simulink model "realtimeBalrob"  (R2024b)
settings: Solver=FixedStepDiscrete  StartTime=0.0  StopTime=50  FixedStep=0.01  RelTol=1e-3  EnableMultiTasking=on
undefined symbols (not defined in the file): chassis, DiscIntNeverNeededParam, Discrete, drv, feedback, filter, gbox, sens, sIn, Time, wheel
libraries: BalRobTbx_baselib x9, simulink x3, ctrlSharedLib x1
settings Model: ExtModeTrigDuration=2  Creator=priesmaxim  LastModifiedBy=priesmaxim
settings SolverCC: AutoInsertRateTranBlk=on
settings OptimizationCC: EnhancedBackFolding=on  PassReuseOutputArgsAs=Individual arguments  ZeroExternalMemoryAtStartup=off  ZeroInternalMemoryAtStartup=off  MaxStackSize=64  OptimizeBlockOrder=speed  DifferentSizesBufferReuse=on  OptimizationCustomize=off  EfficientTunableParamExpr=on
settings DebuggingCC: ParameterTunabilityLossMsg=error
settings HardwareCC: ProdBitPerInt=16  ProdBitPerPointer=16  ProdBitPerSizeT=16  ProdBitPerPtrDiffT=16  ProdLargestAtomicFloat=None  ProdWordSize=8  ProdHWDeviceType=Atmel->AVR
settings SFSimCC: MATLABDynamicMemAlloc=off
settings RTWCC: Description=Embedded Coder  SystemTargetFile=ert.tlc  HardwareBoard=Arduino Mega 2560  TemplateMakefile=ert_default_tmf  Toolchain=Arduino AVR  BuildConfiguration=Faster Runs
settings CodeAppCC: ForceParamTrailComments=on  IgnoreCustomStorageClasses=off  OperatorAnnotations=on  SimulinkDataObjDesc=on  SFDataObjDesc=on  InsertBlockDesc=on
settings ERTTargetCC: SupportContinuousTime=on  SupportVariableSizeSignals=on  ExtModeTransport=3  ExtModeStaticAlloc=on  ExtModeAutomaticAllocSize=off  ExtModeStaticAllocSize=2048  ExtModeMexFile=ext_xcp  ExtModeIntrfLevel=Level2 - Open  InlinedParameterPlacement=Hierarchical

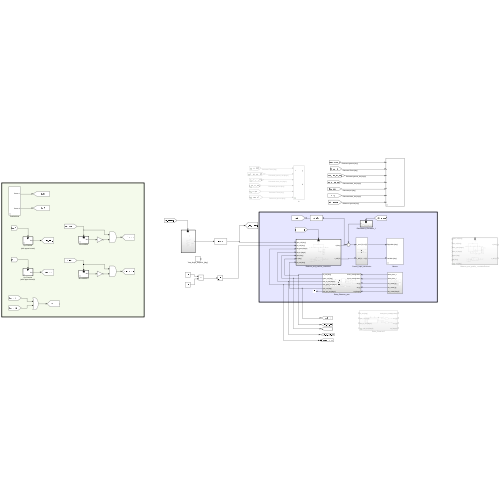
[thumbnail: Simulink's stored preview of the top-level diagram]
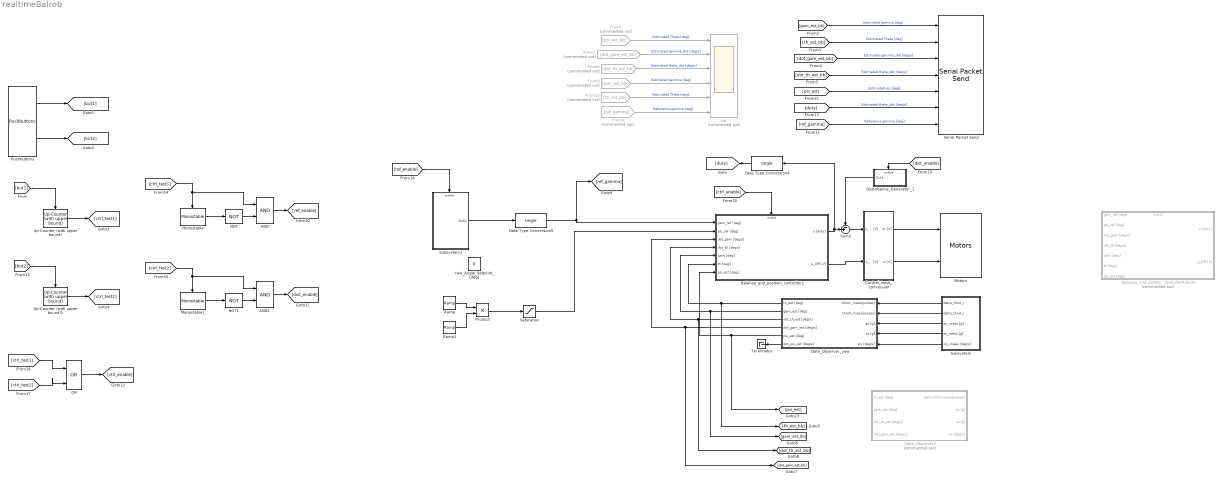
== system realtimeBalrob ==
  AND : Logic  IconShape=distinctive  AllPortsSameDT=off  OutDataTypeStr=boolean
  AND1 : Logic  IconShape=distinctive  AllPortsSameDT=off  OutDataTypeStr=boolean
  Balance_and_positio_ controllerRobust : Subsystem  Commented=on
  Balance_and_position_controller1 : Subsystem
  Control_Input_conversion : Subsystem
  Data Type Conversion4 : DataTypeConversion  OutDataTypeStr=single  SaturateOnIntegerOverflow=off  RndMeth=Floor
  Data Type Conversion5 : DataTypeConversion  OutDataTypeStr=single  SaturateOnIntegerOverflow=off  RndMeth=Floor
  Disturbance_Generator_1 : Subsystem  TreatAsAtomicUnit=on
  From1 : From  Commented=on  GotoTag=psi_est_bb
  From10 : From  Commented=on  GotoTag=th_est_bb
  From6 : From  Commented=on  GotoTag=ref_gamma
  From7 : From  Commented=on  GotoTag=dot_gam_est_bb
  From8 : From  Commented=on  GotoTag=dot_th_est_bb
  From9 : From  Commented=on  GotoTag=gam_est_bb
  Monostable : BalRobTbx_baselib/Utilities/Monostable  Tp=1
      settings: SourceProductName=Balancing Robot Toolbox
  Monostable1 : BalRobTbx_baselib/Utilities/Monostable  Tp=1
      settings: SourceProductName=Balancing Robot Toolbox
  Motors : BalRobTbx_baselib/Outputs/Motors
      settings: SourceProductName=Balancing Robot Toolbox
  NOT : Logic  Operator=NOT  IconShape=distinctive  AllPortsSameDT=off  OutDataTypeStr=boolean
  NOT1 : Logic  Operator=NOT  IconShape=distinctive  AllPortsSameDT=off  OutDataTypeStr=boolean
  OR : Logic  Operator=OR  IconShape=distinctive  AllPortsSameDT=off  OutDataTypeStr=boolean
  Product : Product
  Pushbuttons : BalRobTbx_baselib/Inputs/Pushbuttons
      settings: SourceProductName=Balancing Robot Toolbox
  Ramp : simulink/Sources/Ramp  slope=100  start=0  InitialOutput=0
  Ramp1 : simulink/Sources/Ramp  slope=100  start=0  InitialOutput=0
  Saturation : Saturate  UpperLimit=500  LowerLimit=0
  Serial Packet Send : BalRobTbx_baselib/Communication/Serial Packet Send  serialLinkOpt=Bluetooth  baudRateOpt=38400  waitHostTxCmd=on  txStartCmd=65  txStopCmd=66  packetSpec={'single', 'single', 'single', 'single', 'single', 'single', 'single'}  cobsEncoded=on  nullTerminated=on  showEnablePort=off
      settings: SourceProductName=Balancing Robot Toolbox
  State_Observer2 : Subsystem  Commented=on
  State_Observer_yaw : Subsystem
  Subsystem : Subsystem
  Subsystem1 : Subsystem
  Sum2 : Sum  Inputs=-+|
  Terminator : Terminator
  Up-Counter (with upper bound) : BalRobTbx_baselib/Utilities/Up-Counter (with upper bound)  CMAX=1  C0=0
      settings: SourceProductName=Balancing Robot Toolbox
  Up-Counter (with upper bound)1 : BalRobTbx_baselib/Utilities/Up-Counter (with upper bound)  CMAX=1  C0=0
      settings: SourceProductName=Balancing Robot Toolbox
  Yaw_Angle_Setpoint_[deg] : Constant  Value=0
  bb : Scope  Commented=on  NumInputPorts=6
  wires:
  Control_Input_conversion/1(ur [V]) -> Motors/1
  Sum2/1 -> Control_Input_conversion/1(u_sum [V])
  From10/1 -> bb/5  "Estimated Theta [deg]"
  Disturbance_Generator_1/1(Out1) -> Sum2/1
  From8/1 -> bb/3  "Estimated theta_dot [deg/s]"
  From1/1 -> bb/1  "Estimated Theta [deg]"
  Control_Input_conversion/2(ul [V]) -> Motors/2
  From6/1 -> bb/6  "Reference gamma [deg]"
  From9/1 -> bb/4  "Estimated gamma [deg]"
  [dist_enable] -> Disturbance_Generator_1/Enable
  From7/1 -> bb/2  "Estimated gamma_dot [deg/s]"
  State_Observer_yaw/1(th_est [deg]) -> Balance_and_position_controller1/6(th [deg]), [th_est_bb]
  State_Observer_yaw/2(gam_est [deg]) -> Balance_and_position_controller1/5(gam [deg]), [gam_est_bb]
  State_Observer_yaw/3(dot_th_est [deg/s]) -> Balance_and_position_controller1/4(dot_th [deg/s]), [dot_th_est_bb]
  State_Observer_yaw/4(dot_gam_est [deg/s]) -> [dot_gam_est_bb], Balance_and_position_controller1/3(dot_gam [deg/s])
  [gam_est_bb] -> Serial Packet Send/1  "Estimated gamma [deg]"
  [th_est_bb] -> Serial Packet Send/2  "Estimated Theta [deg]"
  [dot_gam_est_bb] -> Serial Packet Send/3  "Estimated gamma_dot [deg/s]"
  [dot_th_est_bb] -> Serial Packet Send/4  "Estimated theta_dot [deg/s]"
  Data Type Conversion5/1 -> Balance_and_position_controller1/1(gam_ref [deg]), [ref_gamma]
  Data Type Conversion4/1 -> [duty]
  Pushbuttons/1 -> [but1]
  Pushbuttons/2 -> [but2]
  [but1] -> Up-Counter (with upper bound)/Trigger
  Up-Counter (with upper bound)/1 -> [ctrl_test1]
  [but2] -> Up-Counter (with upper bound)1/Trigger
  Up-Counter (with upper bound)1/1 -> [ctrl_test2]
  [ctrl_test1] -> Monostable/Enable, AND/1
  Monostable/1 -> NOT/1
  NOT/1 -> AND/2
  AND/1 -> [ref_enable]
  AND1/1 -> [dist_enable]
  NOT1/1 -> AND1/2
  Monostable1/1 -> NOT1/1
  [ctrl_test2] -> AND1/1, Monostable1/Enable
  [ctrl_test1] -> OR/1
  [ctrl_test2] -> OR/2
  OR/1 -> [ctrl_enable]
  Subsystem1/1(Out1) -> Data Type Conversion5/1
  [ref_enable] -> Subsystem1/Enable
  State_Observer_yaw/6(dot_psi_est [deg/s]) -> Terminator/1
  State_Observer_yaw/5(psi_est [deg]) -> Balance_and_position_controller1/7(psi_est [deg]), [psi_est]
  Subsystem/5(wy_meas [deg/s]) -> State_Observer_yaw/5(wy [deg/s])
  Subsystem/4(az_meas [g]) -> State_Observer_yaw/4(az [g])
  Subsystem/3(ax_meas [g]) -> State_Observer_yaw/3(ax [g])
  Subsystem/2(delta_throt_l) -> State_Observer_yaw/2(throtl_meas[pulses])
  Subsystem/1(delta_throt_r) -> State_Observer_yaw/1(throtr_meas[pulses])
  [duty] -> Serial Packet Send/6  "Estimated theta_dot [deg/s]"
  [ref_gamma] -> Serial Packet Send/7  "Reference gamma [deg]"
  [psi_est] -> Serial Packet Send/5  "Estimated psi [deg]"
  [ctrl_enable] -> Balance_and_position_controller1/Enable
  Balance_and_position_controller1/1(u [duty]) -> Data Type Conversion4/1, Sum2/2
  Balance_and_position_controller1/2(u_diff [V]) -> Control_Input_conversion/2(u_diff [V])
  Ramp/1 -> Product/1
  Ramp1/1 -> Product/2
  Product/1 -> Saturation/1
  Saturation/1 -> Balance_and_position_controller1/2(psi_ref [deg])

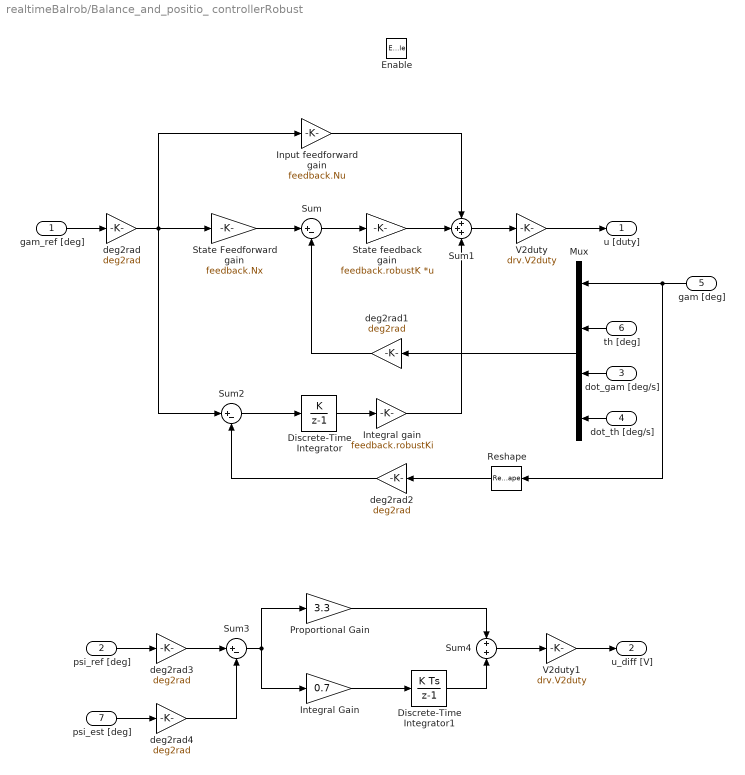
== system realtimeBalrob/Balance_and_positio_ controllerRobust ==
  gam_ref [deg] : Inport
  psi_ref [deg] : Inport  Port=2
  dot_gam [deg/s] : Inport  Port=3
  dot_th [deg/s] : Inport  Port=4
  gam [deg] : Inport  Port=5
  th [deg] : Inport  Port=6
  psi_est [deg] : Inport  Port=7
  Enable : EnablePort
  Discrete-Time Integrator : DiscreteIntegrator  IntegratorMethod=Accumulation: Forward Euler  SampleTime=sIn.Ts  ICPrevOutput=DiscIntNeverNeededParam  ICPrevScaledInput=DiscIntNeverNeededParam
  Discrete-Time Integrator1 : DiscreteIntegrator  SampleTime=-1  ICPrevOutput=DiscIntNeverNeededParam  ICPrevScaledInput=DiscIntNeverNeededParam
  Input feedforward gain : Gain  Gain=feedback.Nu
  Integral Gain : Gain  Gain=0.7
  "Integral gain " : Gain  Gain=feedback.robustKi
  Mux : Mux
  Proportional Gain : Gain  Gain=3.3
  Reshape : Reshape  OutputDimensionality=Customize  OutputDimensions=1
  State Feedforward gain : Gain  Gain=feedback.Nx
  State feedback gain : Gain  Gain=feedback.robustK  Multiplication=Matrix(K*u)
  Sum : Sum  Inputs=|+-
  Sum1 : Sum  Inputs=+++
  Sum2 : Sum  Inputs=|+-
  Sum3 : Sum  Inputs=|+-
  Sum4 : Sum  Inputs=+|+
  V2duty : Gain  Gain=drv.V2duty
  V2duty1 : Gain  Gain=drv.V2duty
  deg2rad{,1..4} (5 alike) : Gain  Gain=deg2rad
  u [duty] : Outport  OutputWhenDisabled=reset  InitialOutput=0
  u_diff [V] : Outport  Port=2  OutputWhenDisabled=reset  InitialOutput=0
  wires:
  gam_ref [deg]/1 -> deg2rad/1
  State Feedforward gain/1 -> Sum/1
  deg2rad1/1 -> Sum/2
  Mux/1 -> deg2rad1/1
  dot_th [deg/s]/1 -> Mux/4
  dot_gam [deg/s]/1 -> Mux/3
  th [deg]/1 -> Mux/2
  Sum/1 -> State feedback gain/1
  State feedback gain/1 -> Sum1/2
  Input feedforward gain/1 -> Sum1/1
  Sum1/1 -> V2duty/1
  V2duty/1 -> u [duty]/1
  Sum2/1 -> Discrete-Time Integrator/1
  deg2rad2/1 -> Sum2/2
  deg2rad/1 -> Sum2/1, Input feedforward gain/1, State Feedforward gain/1
  gam [deg]/1 -> Reshape/1, Mux/1
  Discrete-Time Integrator/1 -> "Integral gain "/1
  Reshape/1 -> deg2rad2/1
  "Integral gain "/1 -> Sum1/3
  Integral Gain/1 -> Discrete-Time Integrator1/1
  Proportional Gain/1 -> Sum4/1
  Sum3/1 -> Integral Gain/1, Proportional Gain/1
  deg2rad3/1 -> Sum3/1
  deg2rad4/1 -> Sum3/2
  Discrete-Time Integrator1/1 -> Sum4/2
  V2duty1/1 -> u_diff [V]/1
  psi_ref [deg]/1 -> deg2rad3/1
  Sum4/1 -> V2duty1/1
  psi_est [deg]/1 -> deg2rad4/1

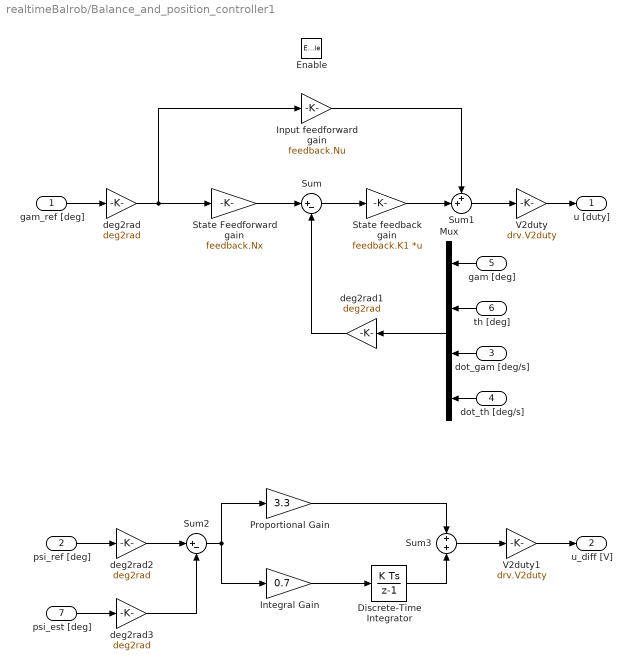
== system realtimeBalrob/Balance_and_position_controller1 ==
  gam_ref [deg] : Inport
  psi_ref [deg] : Inport  Port=2
  dot_gam [deg/s] : Inport  Port=3
  dot_th [deg/s] : Inport  Port=4
  gam [deg] : Inport  Port=5
  th [deg] : Inport  Port=6
  psi_est [deg] : Inport  Port=7
  Enable : EnablePort
  Discrete-Time Integrator : DiscreteIntegrator  SampleTime=-1  ICPrevOutput=DiscIntNeverNeededParam  ICPrevScaledInput=DiscIntNeverNeededParam
  Input feedforward gain : Gain  Gain=feedback.Nu
  Integral Gain : Gain  Gain=0.7
  Mux : Mux
  Proportional Gain : Gain  Gain=3.3
  State Feedforward gain : Gain  Gain=feedback.Nx
  State feedback gain : Gain  Gain=feedback.K1  Multiplication=Matrix(K*u)
  Sum : Sum  Inputs=|+-
  Sum1 : Sum  Inputs=++|
  Sum2 : Sum  Inputs=|+-
  Sum3 : Sum  Inputs=+|+
  V2duty : Gain  Gain=drv.V2duty
  V2duty1 : Gain  Gain=drv.V2duty
  deg2rad{,1..3} (4 alike) : Gain  Gain=deg2rad
  u [duty] : Outport  OutputWhenDisabled=reset  InitialOutput=0
  u_diff [V] : Outport  Port=2  OutputWhenDisabled=reset  InitialOutput=0
  wires:
  gam_ref [deg]/1 -> deg2rad/1
  deg2rad/1 -> Input feedforward gain/1, State Feedforward gain/1
  State Feedforward gain/1 -> Sum/1
  deg2rad1/1 -> Sum/2
  Mux/1 -> deg2rad1/1
  gam [deg]/1 -> Mux/1
  dot_th [deg/s]/1 -> Mux/4
  dot_gam [deg/s]/1 -> Mux/3
  th [deg]/1 -> Mux/2
  Sum/1 -> State feedback gain/1
  State feedback gain/1 -> Sum1/2
  Input feedforward gain/1 -> Sum1/1
  Sum1/1 -> V2duty/1
  V2duty/1 -> u [duty]/1
  psi_ref [deg]/1 -> deg2rad2/1
  psi_est [deg]/1 -> deg2rad3/1
  deg2rad2/1 -> Sum2/1
  deg2rad3/1 -> Sum2/2
  Integral Gain/1 -> Discrete-Time Integrator/1
  Sum2/1 -> Integral Gain/1, Proportional Gain/1
  Proportional Gain/1 -> Sum3/1
  Discrete-Time Integrator/1 -> Sum3/2
  Sum3/1 -> V2duty1/1
  V2duty1/1 -> u_diff [V]/1

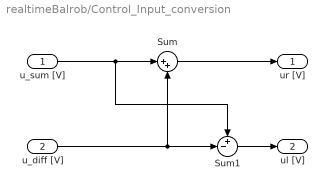
== system realtimeBalrob/Control_Input_conversion ==
  u_sum [V] : Inport
  u_diff [V] : Inport  Port=2
  Sum : Sum  Inputs=|++
  Sum1 : Sum  Inputs=+-|
  ur [V] : Outport
  ul [V] : Outport  Port=2
  wires:
  u_sum [V]/1 -> Sum/1, Sum1/1
  Sum/1 -> ur [V]/1
  u_diff [V]/1 -> Sum/2, Sum1/2
  Sum1/1 -> ul [V]/1

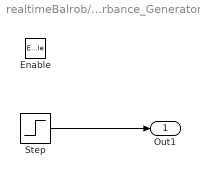
== system realtimeBalrob/Disturbance_Generator_1 ==
  Enable : EnablePort
  Step : Step  Time=10  After=5/drv.duty2V  SampleTime=0
  Out1 : Outport  OutputWhenDisabled=reset  InitialOutput=0
  wires:
  Step/1 -> Out1/1

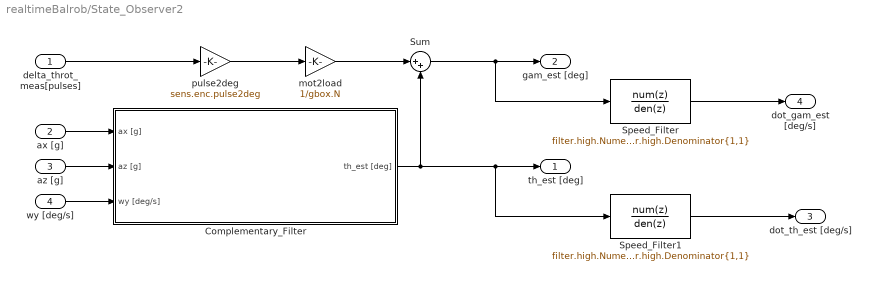
== system realtimeBalrob/State_Observer2 ==
  delta_throt_meas[pulses] : Inport
  ax [g] : Inport  Port=2
  az [g] : Inport  Port=3
  wy [deg/s] : Inport  Port=4
  Complementary_Filter : Subsystem
  Speed_Filter : DiscreteFilter  Numerator=filter.high.Numerator{1,1}  Denominator=filter.high.Denominator{1,1}
  Speed_Filter1 : DiscreteFilter  Numerator=filter.high.Numerator{1,1}  Denominator=filter.high.Denominator{1,1}
  Sum : Sum  Inputs=|++
  mot2load : Gain  Gain=1/gbox.N
  pulse2deg : Gain  Gain=sens.enc.pulse2deg
  th_est [deg] : Outport
  gam_est [deg] : Outport  Port=2
  dot_th_est [deg/s] : Outport  Port=3
  dot_gam_est [deg/s] : Outport  Port=4
  wires:
  wy [deg/s]/1 -> Complementary_Filter/3(wy [deg/s])
  az [g]/1 -> Complementary_Filter/2(az [g])
  ax [g]/1 -> Complementary_Filter/1(ax [g])
  Complementary_Filter/1(th_est [deg]) -> Sum/2, Speed_Filter1/1, th_est [deg]/1
  delta_throt_meas[pulses]/1 -> pulse2deg/1
  pulse2deg/1 -> mot2load/1
  mot2load/1 -> Sum/1
  Sum/1 -> Speed_Filter/1, gam_est [deg]/1
  Speed_Filter1/1 -> dot_th_est [deg/s]/1
  Speed_Filter/1 -> dot_gam_est [deg/s]/1

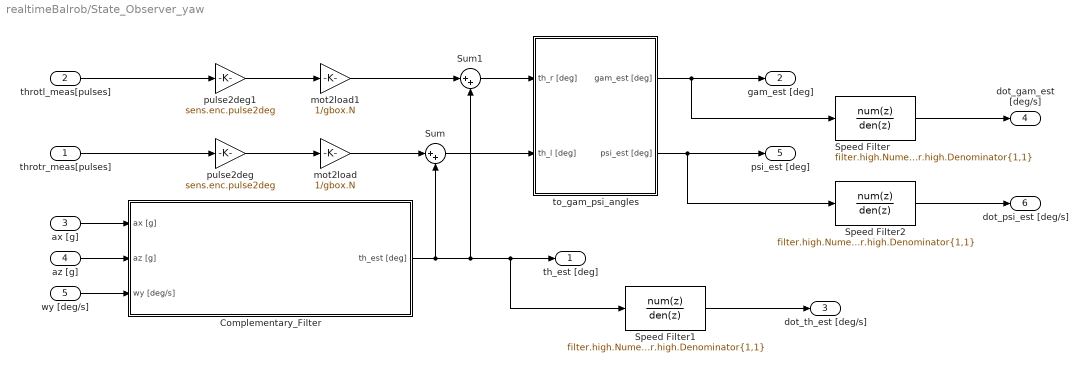
== system realtimeBalrob/State_Observer_yaw ==
  throtr_meas[pulses] : Inport
  throtl_meas[pulses] : Inport  Port=2
  ax [g] : Inport  Port=3
  az [g] : Inport  Port=4
  wy [deg/s] : Inport  Port=5
  Complementary_Filter : Subsystem
  Speed Filter : DiscreteFilter  Numerator=filter.high.Numerator{1,1}  Denominator=filter.high.Denominator{1,1}
  Speed Filter1 : DiscreteFilter  Numerator=filter.high.Numerator{1,1}  Denominator=filter.high.Denominator{1,1}
  Speed Filter2 : DiscreteFilter  Numerator=filter.high.Numerator{1,1}  Denominator=filter.high.Denominator{1,1}
  Sum : Sum  Inputs=|++
  Sum1 : Sum  Inputs=|++
  mot2load : Gain  Gain=1/gbox.N
  mot2load1 : Gain  Gain=1/gbox.N
  pulse2deg : Gain  Gain=sens.enc.pulse2deg
  pulse2deg1 : Gain  Gain=sens.enc.pulse2deg
  to_gam_psi_angles : Subsystem
  th_est [deg] : Outport
  gam_est [deg] : Outport  Port=2
  dot_th_est [deg/s] : Outport  Port=3
  dot_gam_est [deg/s] : Outport  Port=4
  psi_est [deg] : Outport  Port=5
  dot_psi_est [deg/s] : Outport  Port=6
  wires:
  wy [deg/s]/1 -> Complementary_Filter/3(wy [deg/s])
  az [g]/1 -> Complementary_Filter/2(az [g])
  ax [g]/1 -> Complementary_Filter/1(ax [g])
  Complementary_Filter/1(th_est [deg]) -> Sum/2, Sum1/2, Speed Filter1/1, th_est [deg]/1
  throtr_meas[pulses]/1 -> pulse2deg/1
  pulse2deg/1 -> mot2load/1
  mot2load/1 -> Sum/1
  Speed Filter1/1 -> dot_th_est [deg/s]/1
  Speed Filter/1 -> dot_gam_est [deg/s]/1
  mot2load1/1 -> Sum1/1
  pulse2deg1/1 -> mot2load1/1
  throtl_meas[pulses]/1 -> pulse2deg1/1
  Sum/1 -> to_gam_psi_angles/2(th_l [deg])
  Sum1/1 -> to_gam_psi_angles/1(th_r [deg])
  to_gam_psi_angles/1(gam_est [deg]) -> Speed Filter/1, gam_est [deg]/1
  to_gam_psi_angles/2(psi_est [deg]) -> Speed Filter2/1, psi_est [deg]/1
  Speed Filter2/1 -> dot_psi_est [deg/s]/1

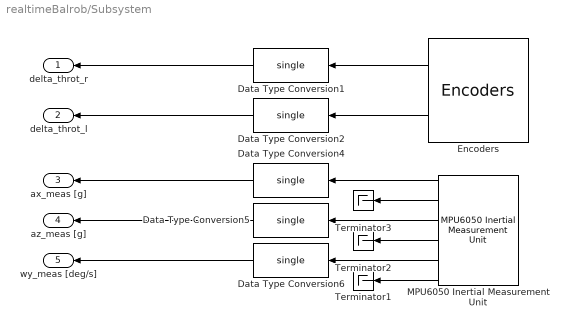
== system realtimeBalrob/Subsystem ==
  Data Type Conversion{1..2,4..6} (5 alike) : DataTypeConversion  OutDataTypeStr=single  SaturateOnIntegerOverflow=off  RndMeth=Floor
  Encoders : BalRobTbx_baselib/Inputs/Encoders
      settings: SourceProductName=Balancing Robot Toolbox
  MPU6050 Inertial Measurement Unit : BalRobTbx_baselib/Inputs/MPU6050 Inertial Measurement Unit
      settings: SourceProductName=Balancing Robot Toolbox
  Terminator1 : Terminator
  Terminator2 : Terminator
  Terminator3 : Terminator
  delta_throt_r : Outport
  delta_throt_l : Outport  Port=2
  ax_meas [g] : Outport  Port=3
  az_meas [g] : Outport  Port=4
  wy_meas [deg/s] : Outport  Port=5
  wires:
  Data Type Conversion6/1 -> wy_meas [deg/s]/1
  MPU6050 Inertial Measurement Unit/6 -> Terminator1/1
  MPU6050 Inertial Measurement Unit/2 -> Terminator3/1
  MPU6050 Inertial Measurement Unit/4 -> Terminator2/1
  Data Type Conversion4/1 -> ax_meas [g]/1
  MPU6050 Inertial Measurement Unit/1 -> Data Type Conversion4/1
  MPU6050 Inertial Measurement Unit/5 -> Data Type Conversion6/1
  MPU6050 Inertial Measurement Unit/3 -> Data Type Conversion5/1
  Data Type Conversion5/1 -> az_meas [g]/1
  Encoders/1 -> Data Type Conversion1/1
  Data Type Conversion1/1 -> delta_throt_r/1
  Encoders/2 -> Data Type Conversion2/1
  Data Type Conversion2/1 -> delta_throt_l/1

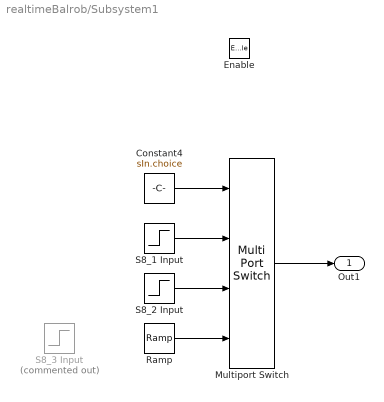
== system realtimeBalrob/Subsystem1 ==
  Enable : EnablePort
  Constant4 : Constant  Value=sIn.choice
  Multiport Switch : MultiPortSwitch  SaturateOnIntegerOverflow=off  InputSameDT=off
  Ramp : simulink/Sources/Ramp  slope=0  start=0  InitialOutput=0
  S8_1 Input : Step  Time=0  After=0  SampleTime=0
  S8_2 Input : Step  Time=0  After=(0.1/wheel.r) *rad2deg  SampleTime=0
  S8_3 Input : Step  Commented=on  Time=0  After=(0.1/wheel.r) *rad2deg  SampleTime=0
  Out1 : Outport  OutputWhenDisabled=reset  InitialOutput=0
  wires:
  Ramp/1 -> Multiport Switch/4
  S8_2 Input/1 -> Multiport Switch/3
  S8_1 Input/1 -> Multiport Switch/2
  Multiport Switch/1 -> Out1/1
  Constant4/1 -> Multiport Switch/1

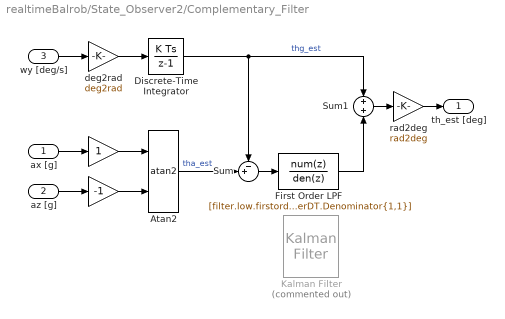
== system realtimeBalrob/State_Observer2/Complementary_Filter ==
  ax [g] : Inport
  az [g] : Inport  Port=2
  wy [deg/s] : Inport  Port=3
  " " : Gain
  "   " : Gain  Gain=-1
  Atan2 : Trigonometry  Operator=atan2
  Discrete-Time Integrator : DiscreteIntegrator  InitialCondition=sIn.x0(2)  SampleTime=sIn.Ts  ICPrevOutput=DiscIntNeverNeededParam  ICPrevScaledInput=DiscIntNeverNeededParam
  First Order LPF : DiscreteTransferFcn  Numerator=[filter.low.firstorderDT.Numerator{1,1}]  Denominator=[filter.low.firstorderDT.Denominator{1,1}]
  Kalman Filter : ctrlSharedLib/Kalman Filter  Commented=on  TimeDomain=Discrete-Time  UseCurrentEstimator=on  ModelSource=LTI State-Space Variable  ModelSourceVariable=ss(0.95,1,1,0,1)  A=0.95  B=1  C=1  D=0  NumberOfStates=1  NumberOfInputs=1  NumberOfOutputs=1  InitialEstimateSource=Dialog  X0=0  P0=10  UseK=off  UseGH=off  NumberOfProcessNoiseInputs=1  G=1  TimeInvariantG=on  H=0  TimeInvariantH=on  Q=0.05  TimeInvariantQ=on  R=1  TimeInvariantR=on  N=0  TimeInvariantN=on  AddInputPort=on  AddEnablePort=off  OutputEstimatedY=off  OutputP=off  Ts=-1
  Sum : Sum  Inputs=-+|
  Sum1 : Sum  Inputs=+|+
  deg2rad : Gain  Gain=deg2rad
  rad2deg : Gain  Gain=rad2deg
  th_est [deg] : Outport
  wires:
  wy [deg/s]/1 -> deg2rad/1
  deg2rad/1 -> Discrete-Time Integrator/1
  az [g]/1 -> "   "/1
  ax [g]/1 -> " "/1
  "   "/1 -> Atan2/2
  " "/1 -> Atan2/1
  Atan2/1 -> Sum/2  "tha_est"
  Discrete-Time Integrator/1 -> Sum1/1, Sum/1  "thg_est"
  Sum/1 -> First Order LPF/1
  First Order LPF/1 -> Sum1/2
  Sum1/1 -> rad2deg/1
  rad2deg/1 -> th_est [deg]/1

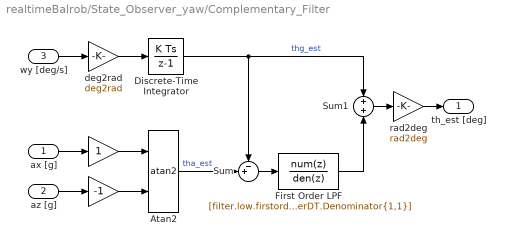
== system realtimeBalrob/State_Observer_yaw/Complementary_Filter ==
  ax [g] : Inport
  az [g] : Inport  Port=2
  wy [deg/s] : Inport  Port=3
  " " : Gain
  "   " : Gain  Gain=-1
  Atan2 : Trigonometry  Operator=atan2
  Discrete-Time Integrator : DiscreteIntegrator  InitialCondition=sIn.x0(2)  SampleTime=sIn.Ts  ICPrevOutput=DiscIntNeverNeededParam  ICPrevScaledInput=DiscIntNeverNeededParam
  First Order LPF : DiscreteTransferFcn  Numerator=[filter.low.firstorderDT.Numerator{1,1}]  Denominator=[filter.low.firstorderDT.Denominator{1,1}]
  Sum : Sum  Inputs=-+|
  Sum1 : Sum  Inputs=+|+
  deg2rad : Gain  Gain=deg2rad
  rad2deg : Gain  Gain=rad2deg
  th_est [deg] : Outport
  wires:
  wy [deg/s]/1 -> deg2rad/1
  deg2rad/1 -> Discrete-Time Integrator/1
  az [g]/1 -> "   "/1
  ax [g]/1 -> " "/1
  "   "/1 -> Atan2/2
  " "/1 -> Atan2/1
  Atan2/1 -> Sum/2  "tha_est"
  Discrete-Time Integrator/1 -> Sum1/1, Sum/1  "thg_est"
  Sum/1 -> First Order LPF/1
  First Order LPF/1 -> Sum1/2
  Sum1/1 -> rad2deg/1
  rad2deg/1 -> th_est [deg]/1

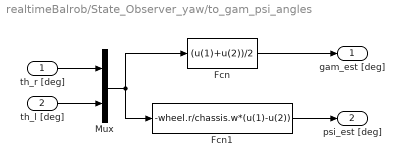
== system realtimeBalrob/State_Observer_yaw/to_gam_psi_angles ==
  th_r [deg] : Inport
  th_l [deg] : Inport  Port=2
  Fcn : Fcn  Expr=(u(1)+u(2))/2
  Fcn1 : Fcn  Expr=-wheel.r/chassis.w*(u(1)-u(2))
  Mux : Mux  Inputs=2
  gam_est [deg] : Outport
  psi_est [deg] : Outport  Port=2
  wires:
  th_r [deg]/1 -> Mux/1
  th_l [deg]/1 -> Mux/2
  Mux/1 -> Fcn1/1, Fcn/1
  Fcn/1 -> gam_est [deg]/1
  Fcn1/1 -> psi_est [deg]/1
